simulink model "CompleteControl_SimpleDC"  (R2023b)
settings: Solver=VariableStepAuto  StartTime=0.0  StopTime=10  RelTol=1e-3
values from neighbouring files (symbols this model uses):
  J = 2.54e-3    (= 0.00254)    [Attitude_OuterLoop.m]    (also in BLDC_measures.m; SystemVariables.m)
  Jb = Js    (= 0.05116)    [Attitude_OuterLoop.m]    (also in SystemVariables.m)
  Js = 0.05116    [Attitude_OuterLoop.m]    (also in BLDC_measures.m; SystemVariables.m)
  Jw = J    (= 0.00254)    [Attitude_OuterLoop.m]    (also in BLDC_measures.m; SystemVariables.m)
  K = place(A,B,p)    [Attitude_OuterLoop.m]    (also in BLDC_measures.m = 11200)
  Ke = 67.5e-3    (= 0.0675)    [Attitude_OuterLoop.m]    (also in BLDC_measures.m; SystemVariables.m)
  Kt = Ke    (= 0.0675)    [Attitude_OuterLoop.m]    (also in BLDC_measures.m; SystemVariables.m)
  Ktt = 78.48e-3    (= 0.07848)    [Attitude_OuterLoop.m]    (also in BLDC_measures.m; SystemVariables.m)
  R = 5.6    [Attitude_OuterLoop.m]    (also in BLDC_measures.m; SystemVariables.m)
libraries: simulink_extras x2, slpidlib x1
settings Model: Creator=Jorge CM  LastModifiedBy=Jorge CM

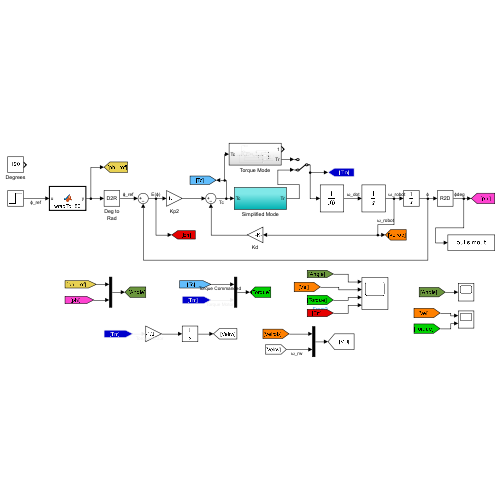
[thumbnail: Simulink's stored preview of the top-level diagram]
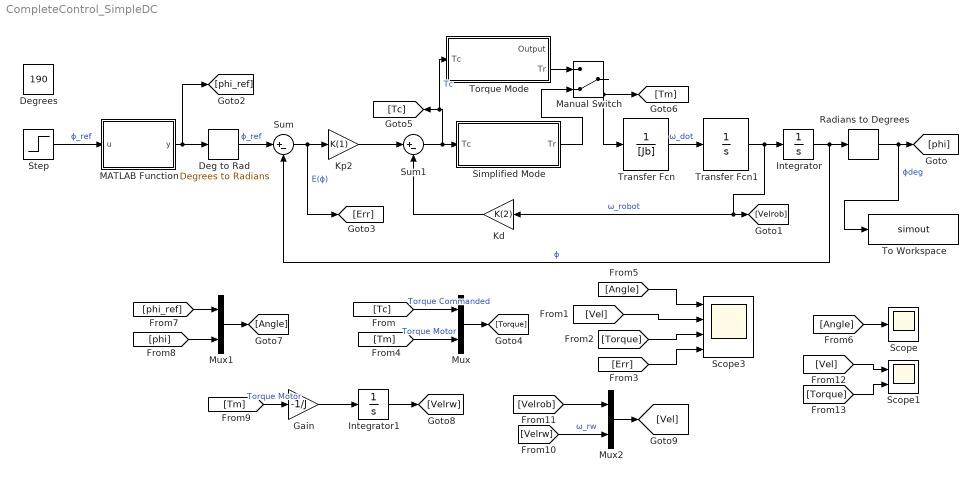
== system CompleteControl_SimpleDC ==
  Deg to Rad : simulink_extras/Transformations/Degrees to Radians
  Degrees : Constant  Value=190
  Gain : Gain  Gain=-1/J
  Integrator : Integrator
  Integrator1 : Integrator
  Kd : Gain  Gain=K(2)
  Kp2 : Gain  Gain=K(1)
  MATLAB Function : MATLAB Function  TreatAsAtomicUnit=on
  Manual Switch : ManualSwitch  CurrentSetting=0
  Mux : Mux  Inputs=2
  Mux1 : Mux  Inputs=2
  Mux2 : Mux  Inputs=2
  Radians to Degrees : simulink_extras/Transformations/Radians to Degrees
  Scope : Scope
  Scope1 : Scope  NumInputPorts=2
  Scope3 : Scope  NumInputPorts=4
  Simplified Mode : Subsystem
  Step : Step  After=170  SampleTime=0
  Sum : Sum  Inputs=|+-
  Sum1 : Sum  Inputs=|+-
  To Workspace : ToWorkspace  VariableName=simout  SaveFormat=Timeseries  SampleTime=-1
      settings: Save2DSignal=2-D array (concatenate along first dimension)
  Torque Mode : Subsystem
  Transfer Fcn : TransferFcn  Denominator=[Jb]
  Transfer Fcn1 : TransferFcn  Denominator=[1 0]
  wires:
  Radians to Degrees/1 -> To Workspace/1, [phi]  "ϕdeg"
  Integrator/1 -> Sum/2, Radians to Degrees/1  "ϕ"
  Deg to Rad/1 -> Sum/1  "ϕ_ref"
  Transfer Fcn/1 -> Transfer Fcn1/1  "ω_dot"
  Sum/1 -> Kp2/1, [Err]  "E(ϕ)"
  Transfer Fcn1/1 -> Integrator/1, [Velrob], Kd/1  "ω_robot"
  [Vel] -> Scope3/2
  Sum1/1 -> Simplified Mode/1(Tc), Torque Mode/1(Tc), [Tc]  "Tc"
  Kd/1 -> Sum1/2
  Kp2/1 -> Sum1/1
  [Tc] -> Mux/1  "Torque Commanded"
  [Tm] -> Mux/2  "Torque Motor"
  Mux/1 -> [Torque]
  [Angle] -> Scope/1
  [phi] -> Mux1/2
  [phi_ref] -> Mux1/1
  Mux1/1 -> [Angle]
  Step/1 -> MATLAB Function/1(u)  "ϕ_ref"
  MATLAB Function/1(y) -> [phi_ref], Deg to Rad/1
  [Tm] -> Gain/1  "Torque Motor"
  Gain/1 -> Integrator1/1
  Integrator1/1 -> [Velrw]
  [Velrw] -> Mux2/2  "ω_rw"
  [Velrob] -> Mux2/1
  Mux2/1 -> [Vel]
  [Angle] -> Scope3/1
  [Torque] -> Scope3/3
  [Err] -> Scope3/4
  [Vel] -> Scope1/1
  [Torque] -> Scope1/2
  Manual Switch/1 -> [Tm], Transfer Fcn/1
  Simplified Mode/1(Tr) -> Manual Switch/2
  Torque Mode/2(Tr) -> Manual Switch/1

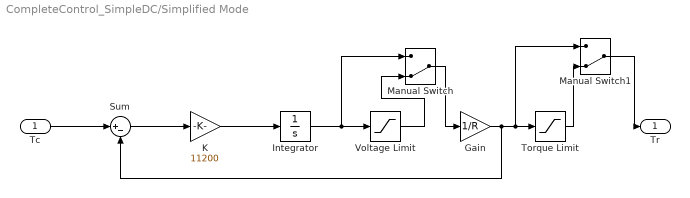
== system CompleteControl_SimpleDC/Simplified Mode ==
  Tc : Inport
  Gain : Gain  Gain=1/R
  Integrator : Integrator
  K : Gain  Gain=11200
  Manual Switch : ManualSwitch  CurrentSetting=0
  Manual Switch1 : ManualSwitch  CurrentSetting=0
  Sum : Sum  Inputs=|+-
  Torque Limit : Saturate  UpperLimit=Ktt  LowerLimit=-Ktt
  Voltage Limit : Saturate  UpperLimit=11  LowerLimit=-11
  Tr : Outport
  wires:
  Tc/1 -> Sum/1
  Sum/1 -> K/1
  K/1 -> Integrator/1
  Gain/1 -> Sum/2, Manual Switch1/1, Torque Limit/1
  Integrator/1 -> Manual Switch/1, Voltage Limit/1
  Manual Switch/1 -> Gain/1
  Voltage Limit/1 -> Manual Switch/2
  Manual Switch1/1 -> Tr/1
  Torque Limit/1 -> Manual Switch1/2

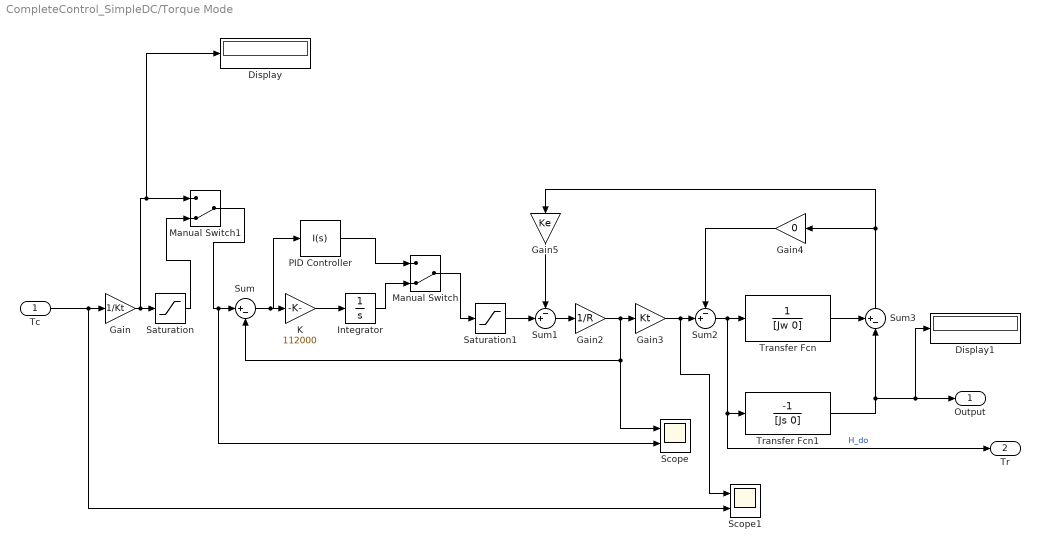
== system CompleteControl_SimpleDC/Torque Mode ==
  Tc : Inport
  Display : Display
  Display1 : Display
  Gain : Gain  Gain=1/Kt
  Gain2 : Gain  Gain=1/R
  Gain3 : Gain  Gain=Kt
  Gain4 : Gain  Gain=0
  Gain5 : Gain  Gain=Ke
  Integrator : Integrator
  K : Gain  Gain=112000
  Manual Switch : ManualSwitch  CurrentSetting=0
  Manual Switch1 : ManualSwitch  CurrentSetting=0
  PID Controller : slpidlib/PID Controller  Controller=I  Form=Parallel  TimeDomain=Continuous-time  UseExternalTs=off  SampleTime=-1  IntegratorMethod=Forward Euler  FilterMethod=Forward Euler  ControllerParametersSource=internal  P=1  I=1120.00158265711  UseKiTs=off  D=0  N=100  UseFilter=on  TunerSelectOption=Transfer Function Based (PID Tuner App)  InitialConditionSource=internal  InitialConditionForIntegrator=0  InitialConditionForFilter=0  DifferentiatorICPrevScaledInput=0  ExternalReset=none  TrackingMode=off  Kt=1  LimitOutput=off  SatLimitsSource=internal  UpperSaturationLimit=inf  LowerSaturationLimit=-inf  LinearizeAsGain=on  AntiWindupMode=none  Kb=1  LimitIntegrator=off  UpperIntegratorSaturationLimit=inf  LowerIntegratorSaturationLimit=-inf  POutMin=[]  POutMax=[]  IOutMin=[]  IOutMax=[]  DOutMin=[]  DOutMax=[]  NOutMin=[]  NOutMax=[]  SumOutMin=[]  SumOutMax=[]  SaturationOutMin=[]  SaturationOutMax=[]  PParamMin=[]  PParamMax=[]  IParamMin=[]  IParamMax=[]  DParamMin=[]  DParamMax=[]  NParamMin=[]  NParamMax=[]  KbParamMin=[]  KbParamMax=[]  KtParamMin=[]  KtParamMax=[]  KbOutMin=[]  KbOutMax=[]  KtOutMin=[]  KtOutMax=[]  IntegratorOutMin=[]  IntegratorOutMax=[]  FilterOutMin=[]  FilterOutMax=[]  SumI1OutMin=[]  SumI1OutMax=[]  SumI2OutMin=[]  SumI2OutMax=[]  SumI3OutMin=[]  SumI3OutMax=[]  SumI4OutMin=[]  SumI4OutMax=[]  SumDOutMin=[]  SumDOutMax=[]  DifferentiatorOutMin=[]  DifferentiatorOutMax=[]  FilterDiffOutCoefMin=[]  FilterDiffOutCoefMax=[]  ReciprocalOutMin=[]  ReciprocalOutMax=[]  SumDenOutMin=[]  SumDenOutMax=[]  SumNumOutMin=[]  SumNumOutMax=[]  DivideOutMin=[]  DivideOutMax=[]  UdiffTsProdOutMin=[]  UdiffTsProdOutMax=[]  NTsProdOutMin=[]  NTsProdOutMax=[]  UintegralTsProdOutMin=[]  UintegralTsProdOutMax=[]  UngainTsProdOutMin=[]  UngainTsProdOutMax=[]  ClampingZeroOutDataTypeStr=Inherit: Inherit via back propagation  ClampingZeroOutMin=[]  ClampingZeroOutMax=[]  FilterDenConstantOutDataTypeStr=Inherit: Inherit via back propagation  FilterDenConstantOutMin=[]  FilterDenConstantOutMax=[]  PCopyOutDataTypeStr=Inherit: Inherit via back propagation  PCopyOutMin=[]  PCopyOutMax=[]  NCopyOutDataTypeStr=Inherit: Inherit via back propagation  NCopyOutMin=[]  NCopyOutMax=[]  IntegratorContinuousStateAttributes=''  IntegratorStateMustResolveToSignalObject=off  IntegratorRTWStateStorageClass=Auto  FilterContinuousStateAttributes=''  FilterStateMustResolveToSignalObject=off  FilterRTWStateStorageClass=Auto  ParallelPVariant=Disabled  IdealPVariant=Disabled  IVariant=InternalParameters  DVariant=Disabled  IntegratorVariant=Continuous  SatVariant=Disabled  AWVariant=Passthrough  PCopyVariant=Disabled  TRVariant=Disabled  FdbkBlocksVariant=Forward  IdealPFdbkVariant=Disabled  SatFdbkVariant=Disabled  DerivativeFilterVariant=Disabled  NVariant=Disabled  NCopyVariant=Disabled_SignalSpec  FilterICVariant=Disabled  IntegratorICVariant=InternalICs  ExternalResetVariant=Disabled  TRSumVariant=Passthrough  SumFdbkVariant=Disabled  SumVariant=Passthrough_I  TsampFilterVariant=InternalTs  TsampNgainVariant=Passthrough  TsampIntegralVariant=Disabled_SignalSpec  ExternalSaturationOutDataTypeStr=Inherit: Same as second input
  Saturation : Saturate  UpperLimit=1  LowerLimit=-1
  Saturation1 : Saturate  UpperLimit=11  LowerLimit=-11
  Scope : Scope  NumInputPorts=2
  Scope1 : Scope  NumInputPorts=2
  Sum : Sum  Inputs=|+-
  Sum1 : Sum  Inputs=-+|
  Sum2 : Sum  Inputs=-+|
  Sum3 : Sum  Inputs=+-|
  Transfer Fcn : TransferFcn  Denominator=[Jw 0]
  Transfer Fcn1 : TransferFcn  Numerator=[-1]  Denominator=[Js 0]
  Output : Outport
  Tr : Outport  Port=2
  wires:
  PID Controller/1 -> Manual Switch/1
  Tc/1 -> Scope1/2, Gain/1
  Manual Switch1/1 -> Scope/2, Sum/1
  Manual Switch/1 -> Saturation1/1
  Sum3/1 -> Gain5/1, Gain4/1
  Gain4/1 -> Sum2/1
  Integrator/1 -> Manual Switch/2
  Sum1/1 -> Gain2/1
  Sum2/1 -> Tr/1, Transfer Fcn1/1, Transfer Fcn/1  "H_do"
  Transfer Fcn/1 -> Sum3/1
  Gain3/1 -> Scope1/1, Sum2/2
  Saturation/1 -> Manual Switch1/2
  Saturation1/1 -> Sum1/2
  Gain2/1 -> Gain3/1, Scope/1, Sum/2
  Sum/1 -> PID Controller/1, K/1
  K/1 -> Integrator/1
  Gain/1 -> Display/1, Manual Switch1/1, Saturation/1
  Gain5/1 -> Sum1/1
  Transfer Fcn1/1 -> Sum3/2, Display1/1, Output/1

== matlab function CompleteControl_SimpleDC/MATLAB Function ==
  data: u input; y output
function y = wrapTo180(u)
% Función que normaliza un ángulo entre -180 y 180 grados
    y = mod(u + 180, 360) - 180;
end
